simulink model "sampleModel76"  (R2021b)
settings: Solver=VariableStepAuto  StartTime=0.0  StopTime=10.0  RelTol=1e-3
undefined symbols (not defined in the file or in its folder): Newton, Raphson
libraries: simulink x9
settings Model: Creator=user  LastModifiedBy=user

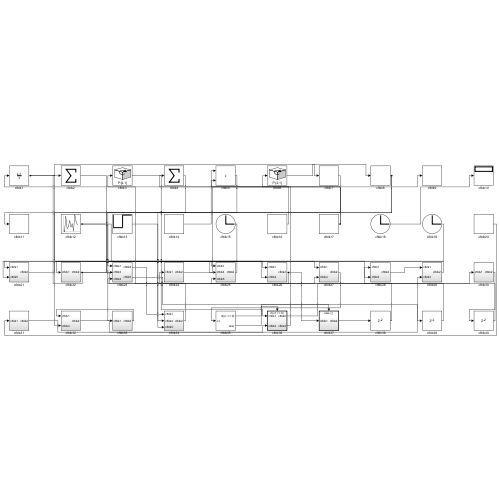
[thumbnail: Simulink's stored preview of the top-level diagram]
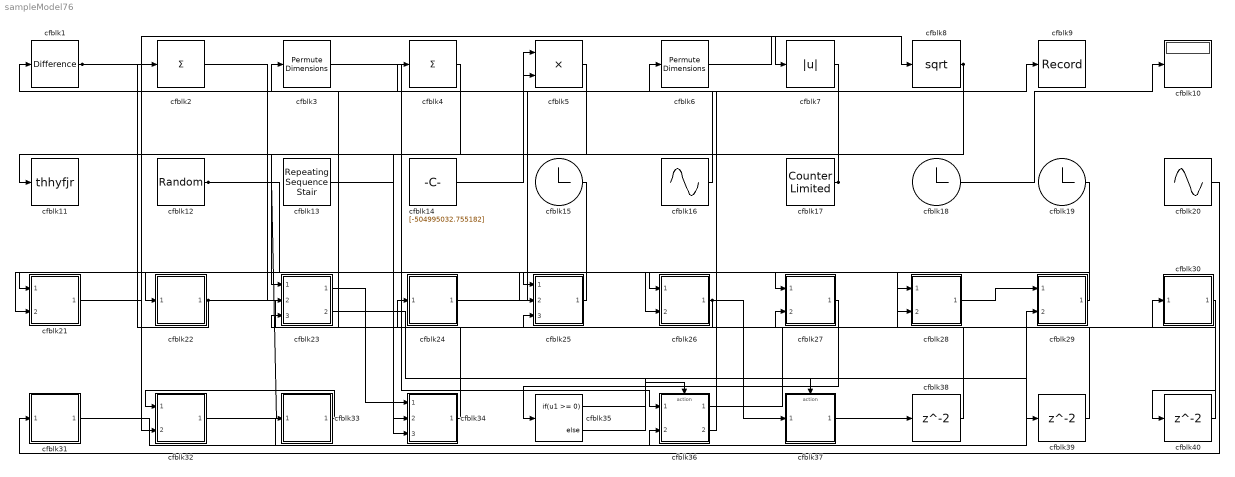
== system sampleModel76 ==
  cfblk1 : simulink/Discrete/Difference  ICPrevInput=0.0  OutMin=[]  OutMax=[]  OutDataTypeStr=Inherit: Inherit via back propagation  OutDataType=fixdt(1, 16)  OutScaling=2^-10  DoSatur=off
  cfblk10 : Display
  cfblk11 : ToWorkspace  VariableName=thhyfjr  SaveFormat=Timeseries  SampleTime=-1
  cfblk12 : UniformRandomNumber  Minimum=[-6258414574.924370]  Maximum=[6831308308.805039]  Seed=[97532044.000000]  SampleTime=0.1
  cfblk13 : simulink/Sources/Repeating Sequence Stair  OutValues=[337847382.557305, 394865707.663621]  tsamp=-1  OutMin=[]  OutMax=[]  OutDataTypeStr=double  OutputDataTypeScalingMode=double  OutDataType=fixdt(0,8)  ConRadixGroup=Best Precision: Vector-wise  OutScaling=2^-12
  cfblk14 : Constant  Value=[-504995032.755182]  SampleTime=1
  cfblk15 : Clock
  cfblk16 : Sin  Amplitude=[553134842.452992]  Bias=[-719838863.569597]  SampleTime=0
  cfblk17 : simulink/Sources/Counter Limited  uplimit=[253.000000]  tsamp=-1
  cfblk18 : Clock
  cfblk19 : Clock
  cfblk2 : Sum  Inputs=+
  cfblk20 : Sin  Amplitude=[114159622.682471]  Bias=[19690642.448085]  SampleTime=0
  cfblk21 : Subsystem
  cfblk22 : Subsystem
  cfblk23 : Subsystem
  cfblk24 : Subsystem
  cfblk25 : Subsystem
  cfblk26 : Subsystem
  cfblk27 : Subsystem
  cfblk28 : Subsystem
  cfblk29 : Subsystem
  cfblk3 : PermuteDimensions
  cfblk30 : Subsystem
  cfblk31 : Subsystem
  cfblk32 : Subsystem
  cfblk33 : Subsystem
  cfblk34 : Subsystem
  cfblk35 : If  IfExpression=u1 >= 0  SampleTime=1
  cfblk36 : Subsystem  TreatAsAtomicUnit=on
  cfblk37 : Subsystem  TreatAsAtomicUnit=on
  cfblk38 : Delay  SampleTime=1
  cfblk39 : Delay  SampleTime=1
  cfblk4 : Sum  Inputs=+
  cfblk40 : Delay  SampleTime=1
  cfblk5 : Product
  cfblk6 : PermuteDimensions
  cfblk7 : Abs
  cfblk8 : Sqrt  SaturateOnIntegerOverflow=on
  cfblk9 : Record  FileSettingsInternal="{\"entries\":[{\"content\":{\"excelSettings\":{\"content\":{},\"type\":\"Streamout.ExcelSettings\"}},\"type\":\"Streamout.FileSettingStorage\",\"uuid\":\"2890a466-a182-4740-b0dd-081fec509c8b\"}],\"packageUris\":[\"http://schema.mathworks.com/mf0/streamout_blocks/R2020a\"],\"version\":\"1.0\"}"  SignalsInternal="{\"entries\":[{\"content\":{\"signals\":[{\"content\":{\"blockPath\":[\"sampleModel76/cfblk9\"],\"channel\":[],\"dimensions\":[1,1],\"domain\":\"sampleModel76/cfblk9\",\"lineColor\":\"#ff13a6\",\"plots\":[1],\"port\":1,\"sid\":[\"\"],\"signalID\":2805,\"signalName\":\"cfblk24\"},\"type\":\"RecordBlkView.Signal\",\"uuid\":\"1ef18046-e972-444f-897b-fd5f1b567179\"}]},\"type\":\"RecordBlkView.InputSignals\",\"uuid\":\"a4c8da73-c598-4369-b845-44db3d8a0e59\"}],\"packageUris\":[\"http://schema.mathworks.com/mf0/streamout_blocks/R2020a\"],\"version\":\"1.0\"}"  VisualizationBindings="{\"sparklinesplugin\":{\"info\":[{\"bindingParametersList\":[],\"subplotID\":1}]}}"
  wires:
  cfblk28/1(cfblk2) -> cfblk29/1(cfblk1)
  cfblk26/1(cfblk2) -> cfblk37/1(cfblk1), cfblk23/3(cfblk4)
  cfblk19/1 -> cfblk22/1(cfblk1)
  cfblk18/1 -> cfblk10/1
  cfblk31/1(cfblk2) -> cfblk29/2(cfblk3)
  cfblk36/1(cfblk2) -> cfblk30/1(cfblk1)
  cfblk24/1(cfblk2) -> cfblk9/1
  cfblk23/1(cfblk2) -> cfblk34/1(cfblk1)
  cfblk20/1 -> cfblk31/1(cfblk1)
  cfblk22/1(cfblk2) -> cfblk2/1, cfblk27/1(cfblk1), cfblk27/2(cfblk4)
  cfblk17/1 -> cfblk5/1, cfblk1/1
  cfblk3/1 -> cfblk36/1(cfblk1)
  cfblk32/1(cfblk2) -> cfblk36/2(cfblk3)
  cfblk1/1 -> cfblk7/1, cfblk28/2(cfblk3)
  cfblk25/1(cfblk2) -> cfblk21/1(cfblk1)
  cfblk15/1 -> cfblk21/2(cfblk5)
  cfblk27/1(cfblk2) -> cfblk35/1
  cfblk12/1 -> cfblk33/1(cfblk1), cfblk26/2(cfblk4)
  cfblk5/1 -> cfblk23/1(cfblk1)
  cfblk16/1 -> cfblk4/1
  cfblk13/1 -> cfblk34/2(cfblk4)
  cfblk7/1 -> cfblk11/1
  cfblk8/1 -> cfblk34/3(cfblk5), cfblk23/2(cfblk3)
  cfblk6/1 -> cfblk8/1
  cfblk29/1(cfblk2) -> cfblk25/1(cfblk1)
  cfblk2/1 -> cfblk25/2(cfblk4)
  cfblk36/2(cfblk4) -> cfblk6/1
  cfblk14/1 -> cfblk5/2
  cfblk33/1(cfblk2) -> cfblk32/1(cfblk1)
  cfblk21/1(cfblk2) -> cfblk26/1(cfblk1)
  cfblk34/1(cfblk2) -> cfblk24/1(cfblk1)
  cfblk4/1 -> cfblk32/2(cfblk4)
  cfblk35/1 -> cfblk36/Action
  cfblk35/2 -> cfblk37/Action
  cfblk37/1(cfblk2) -> cfblk38/1
  cfblk38/1 -> cfblk28/1(cfblk1)
  cfblk23/2(cfblk5) -> cfblk39/1
  cfblk39/1 -> cfblk25/3(cfblk5)
  cfblk30/1(cfblk2) -> cfblk40/1
  cfblk40/1 -> cfblk3/1

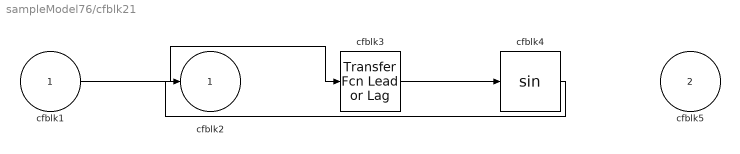
== system sampleModel76/cfblk21 ==
  cfblk1 : Inport
  cfblk5 : Inport  Port=2
  cfblk3 : simulink/Discrete/Transfer Fcn Lead or Lag  PoleZ=0.95  ZeroZ=0.75  ICPrevOutput=0.0  ICPrevInput=0.0  DoSatur=off
      settings: SourceProductBaseCode=SL
  cfblk4 : Trigonometry
  cfblk2 : Outport
  wires:
  cfblk1/1 -> cfblk3/1
  cfblk3/1 -> cfblk4/1
  cfblk4/1 -> cfblk2/1

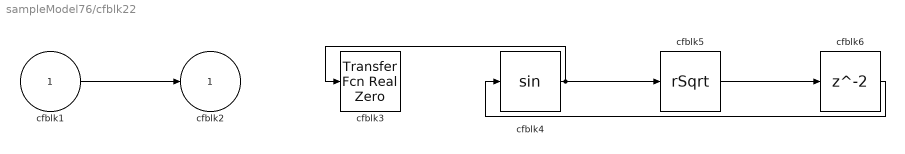
== system sampleModel76/cfblk22 ==
  cfblk1 : Inport
  cfblk3 : simulink/Discrete/Transfer Fcn Real Zero  ZeroZ=0.75  ICPrevInput=0.0  DoSatur=off
      settings: SourceProductBaseCode=SL
  cfblk4 : Trigonometry
  cfblk5 : Sqrt  Operator=rSqrt  AlgorithmType=Newton-Raphson  SaturateOnIntegerOverflow=on
  cfblk6 : Delay  SampleTime=1
  cfblk2 : Outport
  wires:
  cfblk4/1 -> cfblk5/1, cfblk3/1
  cfblk1/1 -> cfblk2/1
  cfblk5/1 -> cfblk6/1
  cfblk6/1 -> cfblk4/1

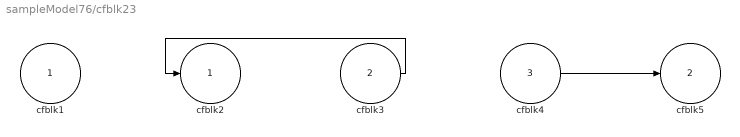
== system sampleModel76/cfblk23 ==
  cfblk1 : Inport
  cfblk3 : Inport  Port=2
  cfblk4 : Inport  Port=3
  cfblk2 : Outport
  cfblk5 : Outport  Port=2
  wires:
  cfblk4/1 -> cfblk5/1
  cfblk3/1 -> cfblk2/1

== system sampleModel76/cfblk24 ==
  cfblk1 : Inport
  cfblk3 : DiscreteFilter  SampleTime=1
  cfblk2 : Outport
  wires:
  cfblk1/1 -> cfblk3/1
  cfblk3/1 -> cfblk2/1

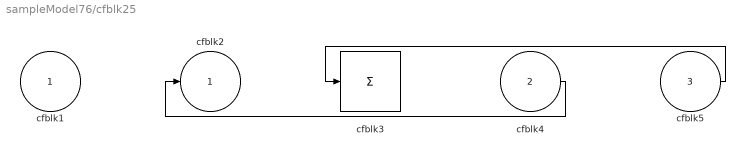
== system sampleModel76/cfblk25 ==
  cfblk1 : Inport
  cfblk4 : Inport  Port=2
  cfblk5 : Inport  Port=3
  cfblk3 : Sum  Inputs=+
  cfblk2 : Outport
  wires:
  cfblk5/1 -> cfblk3/1
  cfblk4/1 -> cfblk2/1

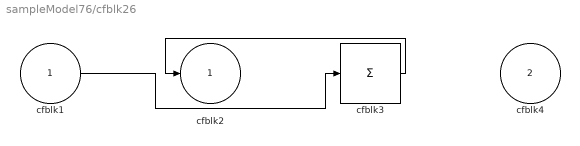
== system sampleModel76/cfblk26 ==
  cfblk1 : Inport
  cfblk4 : Inport  Port=2
  cfblk3 : Sum  Inputs=+
  cfblk2 : Outport
  wires:
  cfblk3/1 -> cfblk2/1
  cfblk1/1 -> cfblk3/1

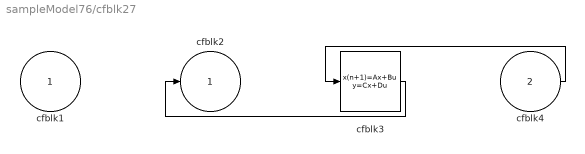
== system sampleModel76/cfblk27 ==
  cfblk1 : Inport
  cfblk4 : Inport  Port=2
  cfblk3 : DiscreteStateSpace
  cfblk2 : Outport
  wires:
  cfblk4/1 -> cfblk3/1
  cfblk3/1 -> cfblk2/1

== system sampleModel76/cfblk28 ==
  cfblk1 : Inport
  cfblk3 : Inport  Port=2
  cfblk2 : Outport
  wires:
  cfblk1/1 -> cfblk2/1

== system sampleModel76/cfblk29 ==
  cfblk1 : Inport
  cfblk3 : Inport  Port=2
  cfblk2 : Outport
  wires:
  cfblk3/1 -> cfblk2/1

== system sampleModel76/cfblk30 ==
  cfblk1 : Inport
  cfblk3 : simulink/Discrete/Difference  ICPrevInput=0.0  OutMin=[]  OutMax=[]  OutDataTypeStr=Inherit: Inherit via back propagation  OutDataType=fixdt(1, 16)  OutScaling=2^-10  DoSatur=off
  cfblk2 : Outport
  wires:
  cfblk1/1 -> cfblk3/1
  cfblk3/1 -> cfblk2/1

== system sampleModel76/cfblk31 ==
  cfblk1 : Inport
  cfblk3 : ComplexToMagnitudeAngle
  cfblk2 : Outport
  wires:
  cfblk1/1 -> cfblk2/1, cfblk3/1

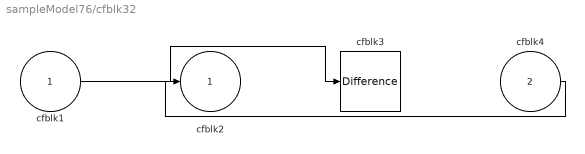
== system sampleModel76/cfblk32 ==
  cfblk1 : Inport
  cfblk4 : Inport  Port=2
  cfblk3 : simulink/Discrete/Difference  ICPrevInput=0.0  OutMin=[]  OutMax=[]  OutDataTypeStr=Inherit: Inherit via back propagation  OutDataType=fixdt(1, 16)  OutScaling=2^-10  DoSatur=off
  cfblk2 : Outport
  wires:
  cfblk1/1 -> cfblk3/1
  cfblk4/1 -> cfblk2/1

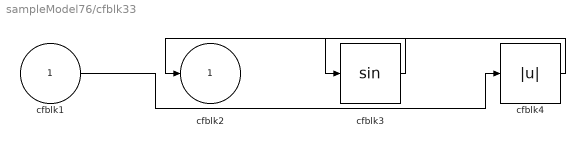
== system sampleModel76/cfblk33 ==
  cfblk1 : Inport
  cfblk3 : Trigonometry
  cfblk4 : Abs
  cfblk2 : Outport
  wires:
  cfblk3/1 -> cfblk2/1
  cfblk1/1 -> cfblk4/1
  cfblk4/1 -> cfblk3/1

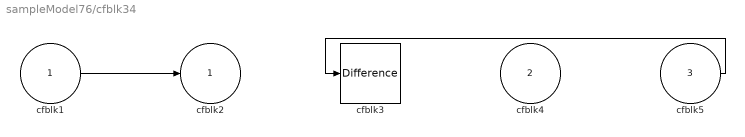
== system sampleModel76/cfblk34 ==
  cfblk1 : Inport
  cfblk4 : Inport  Port=2
  cfblk5 : Inport  Port=3
  cfblk3 : simulink/Discrete/Difference  ICPrevInput=0.0  OutMin=[]  OutMax=[]  OutDataTypeStr=Inherit: Inherit via back propagation  OutDataType=fixdt(1, 16)  OutScaling=2^-10  DoSatur=off
  cfblk2 : Outport
  wires:
  cfblk1/1 -> cfblk2/1
  cfblk5/1 -> cfblk3/1

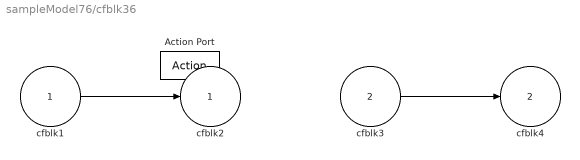
== system sampleModel76/cfblk36 ==
  cfblk1 : Inport
  cfblk3 : Inport  Port=2
  Action Port : ActionPort  ActionPortLabel=if(u1 >= 0)
  cfblk2 : Outport
  cfblk4 : Outport  Port=2
  wires:
  cfblk1/1 -> cfblk2/1
  cfblk3/1 -> cfblk4/1

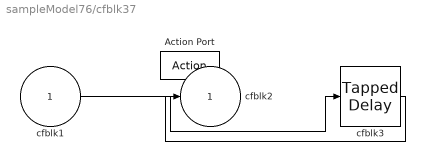
== system sampleModel76/cfblk37 ==
  cfblk1 : Inport
  Action Port : ActionPort  ActionPortLabel=else
  cfblk3 : simulink/Discrete/Tapped Delay  vinit=0.0  samptime=-1  NumDelays=1  DelayOrder=Oldest  includeCurrent=off
  cfblk2 : Outport
  wires:
  cfblk1/1 -> cfblk3/1
  cfblk3/1 -> cfblk2/1
